simulink model "LMS_cs"  (R2023a)
settings: Solver=ode5  StartTime=0.0  StopTime=inf  FixedStep=1/200  RelTol=1e-3
PreLoadFcn:
  | mbxruntime.callbacks.PreLoadFcn(bdroot);
PostLoadFcn:
  | mbxruntime.callbacks.PostLoadFcn(bdroot);
InitFcn:
  | mbxruntime.callbacks.InitFcn(bdroot);
StartFcn:
  | mbxruntime.callbacks.StartFcn(bdroot);
StopFcn:
  | mbxruntime.callbacks.StopFcn(bdroot);
model workspace (MAT data in the model file):
  mbox_table : object (value not decoded)
  model_closed = 0
  sim_status = 0
undefined symbols (not defined in the file or in its folder): DiscIntNeverNeededParam, WheelL0, WheelL1, WheelR0, WheelR1
libraries: simulink x462, simulink_extras x117, PreScanSimulinkLibrary x33, PreScanUsefulBlocks x6, instrumentseriallib x5, simulink_need_slupdate x1
(part 6 of 68)

== system LMS_cs/WheelL0_BMW_X5_SUV_1 ==
  WheelL0_BMW_X5_SUV_1 : Inport  Tag=inport/JointActuator  OutDataTypeStr=Bus: PRESCAN_POSE_DATA  SampleTime=2/200  BusOutputAsStruct=on
  Actuator : Subsystem  Tag=VisuJoint  mask(PreScan Sink Block: VisuJoint){UniqueID=3662, Translate_ObjectID3D=BMW_X5_SUV_1.WheelL0, Rotate_ObjectID3D=BMW_X5_SUV_1.WheelL0, TimeStep=2/200, DisplayName=[]}
      mask prompts: UniqueID "Parent Unique ID"; Translate_ObjectID3D "Translate Object Name"; Rotate_ObjectID3D "Rotate Object Name"; TimeStep "Simulation Step"; DisplayName "Display Name"
      mask help:
      | The VisuJoint block provides a way to adapt the location and orientation of a part of an object.
      |
      | For more information, please click Help.
      settings: DeleteFcn=PreScanBlockDeleteFcn;
      mask Help: eval('openHelp(223)')
      mask Display: image(imread('Joint.png'))
  wires:
  WheelL0_BMW_X5_SUV_1/1 -> Actuator/1(Joint)

== system LMS_cs/WheelL0_BMW_X5_SUV_10 ==
  WheelL0_BMW_X5_SUV_10 : Inport  Tag=inport/JointActuator  OutDataTypeStr=Bus: PRESCAN_POSE_DATA  SampleTime=2/200  BusOutputAsStruct=on
  Actuator : Subsystem  Tag=VisuJoint  mask(PreScan Sink Block: VisuJoint){UniqueID=3671, Translate_ObjectID3D=BMW_X5_SUV_10.WheelL0, Rotate_ObjectID3D=BMW_X5_SUV_10.WheelL0, TimeStep=2/200, DisplayName=[]}
      mask prompts: UniqueID "Parent Unique ID"; Translate_ObjectID3D "Translate Object Name"; Rotate_ObjectID3D "Rotate Object Name"; TimeStep "Simulation Step"; DisplayName "Display Name"
      mask help:
      | The VisuJoint block provides a way to adapt the location and orientation of a part of an object.
      |
      | For more information, please click Help.
      settings: DeleteFcn=PreScanBlockDeleteFcn;
      mask Help: eval('openHelp(223)')
      mask Display: image(imread('Joint.png'))
  wires:
  WheelL0_BMW_X5_SUV_10/1 -> Actuator/1(Joint)

== system LMS_cs/WheelL0_BMW_X5_SUV_11 ==
  WheelL0_BMW_X5_SUV_11 : Inport  Tag=inport/JointActuator  OutDataTypeStr=Bus: PRESCAN_POSE_DATA  SampleTime=2/200  BusOutputAsStruct=on
  Actuator : Subsystem  Tag=VisuJoint  mask(PreScan Sink Block: VisuJoint){UniqueID=3672, Translate_ObjectID3D=BMW_X5_SUV_11.WheelL0, Rotate_ObjectID3D=BMW_X5_SUV_11.WheelL0, TimeStep=2/200, DisplayName=[]}
      mask prompts: UniqueID "Parent Unique ID"; Translate_ObjectID3D "Translate Object Name"; Rotate_ObjectID3D "Rotate Object Name"; TimeStep "Simulation Step"; DisplayName "Display Name"
      mask help:
      | The VisuJoint block provides a way to adapt the location and orientation of a part of an object.
      |
      | For more information, please click Help.
      settings: DeleteFcn=PreScanBlockDeleteFcn;
      mask Help: eval('openHelp(223)')
      mask Display: image(imread('Joint.png'))
  wires:
  WheelL0_BMW_X5_SUV_11/1 -> Actuator/1(Joint)

== system LMS_cs/WheelL0_BMW_X5_SUV_12 ==
  WheelL0_BMW_X5_SUV_12 : Inport  Tag=inport/JointActuator  OutDataTypeStr=Bus: PRESCAN_POSE_DATA  SampleTime=2/200  BusOutputAsStruct=on
  Actuator : Subsystem  Tag=VisuJoint  mask(PreScan Sink Block: VisuJoint){UniqueID=5321, Translate_ObjectID3D=BMW_X5_SUV_12.WheelL0, Rotate_ObjectID3D=BMW_X5_SUV_12.WheelL0, TimeStep=2/200, DisplayName=[]}
      mask prompts: UniqueID "Parent Unique ID"; Translate_ObjectID3D "Translate Object Name"; Rotate_ObjectID3D "Rotate Object Name"; TimeStep "Simulation Step"; DisplayName "Display Name"
      mask help:
      | The VisuJoint block provides a way to adapt the location and orientation of a part of an object.
      |
      | For more information, please click Help.
      settings: DeleteFcn=PreScanBlockDeleteFcn;
      mask Help: eval('openHelp(223)')
      mask Display: image(imread('Joint.png'))
  wires:
  WheelL0_BMW_X5_SUV_12/1 -> Actuator/1(Joint)

== system LMS_cs/WheelL0_BMW_X5_SUV_13 ==
  WheelL0_BMW_X5_SUV_13 : Inport  Tag=inport/JointActuator  OutDataTypeStr=Bus: PRESCAN_POSE_DATA  SampleTime=2/200  BusOutputAsStruct=on
  Actuator : Subsystem  Tag=VisuJoint  mask(PreScan Sink Block: VisuJoint){UniqueID=5322, Translate_ObjectID3D=BMW_X5_SUV_13.WheelL0, Rotate_ObjectID3D=BMW_X5_SUV_13.WheelL0, TimeStep=2/200, DisplayName=[]}
      mask prompts: UniqueID "Parent Unique ID"; Translate_ObjectID3D "Translate Object Name"; Rotate_ObjectID3D "Rotate Object Name"; TimeStep "Simulation Step"; DisplayName "Display Name"
      mask help:
      | The VisuJoint block provides a way to adapt the location and orientation of a part of an object.
      |
      | For more information, please click Help.
      settings: DeleteFcn=PreScanBlockDeleteFcn;
      mask Help: eval('openHelp(223)')
      mask Display: image(imread('Joint.png'))
  wires:
  WheelL0_BMW_X5_SUV_13/1 -> Actuator/1(Joint)

== system LMS_cs/WheelL0_BMW_X5_SUV_2 ==
  WheelL0_BMW_X5_SUV_2 : Inport  Tag=inport/JointActuator  OutDataTypeStr=Bus: PRESCAN_POSE_DATA  SampleTime=2/200  BusOutputAsStruct=on
  Actuator : Subsystem  Tag=VisuJoint  mask(PreScan Sink Block: VisuJoint){UniqueID=3663, Translate_ObjectID3D=BMW_X5_SUV_2.WheelL0, Rotate_ObjectID3D=BMW_X5_SUV_2.WheelL0, TimeStep=2/200, DisplayName=[]}
      mask prompts: UniqueID "Parent Unique ID"; Translate_ObjectID3D "Translate Object Name"; Rotate_ObjectID3D "Rotate Object Name"; TimeStep "Simulation Step"; DisplayName "Display Name"
      mask help:
      | The VisuJoint block provides a way to adapt the location and orientation of a part of an object.
      |
      | For more information, please click Help.
      settings: DeleteFcn=PreScanBlockDeleteFcn;
      mask Help: eval('openHelp(223)')
      mask Display: image(imread('Joint.png'))
  wires:
  WheelL0_BMW_X5_SUV_2/1 -> Actuator/1(Joint)

== system LMS_cs/WheelL0_BMW_X5_SUV_3 ==
  WheelL0_BMW_X5_SUV_3 : Inport  Tag=inport/JointActuator  OutDataTypeStr=Bus: PRESCAN_POSE_DATA  SampleTime=2/200  BusOutputAsStruct=on
  Actuator : Subsystem  Tag=VisuJoint  mask(PreScan Sink Block: VisuJoint){UniqueID=3664, Translate_ObjectID3D=BMW_X5_SUV_3.WheelL0, Rotate_ObjectID3D=BMW_X5_SUV_3.WheelL0, TimeStep=2/200, DisplayName=[]}
      mask prompts: UniqueID "Parent Unique ID"; Translate_ObjectID3D "Translate Object Name"; Rotate_ObjectID3D "Rotate Object Name"; TimeStep "Simulation Step"; DisplayName "Display Name"
      mask help:
      | The VisuJoint block provides a way to adapt the location and orientation of a part of an object.
      |
      | For more information, please click Help.
      settings: DeleteFcn=PreScanBlockDeleteFcn;
      mask Help: eval('openHelp(223)')
      mask Display: image(imread('Joint.png'))
  wires:
  WheelL0_BMW_X5_SUV_3/1 -> Actuator/1(Joint)

== system LMS_cs/WheelL0_BMW_X5_SUV_4 ==
  WheelL0_BMW_X5_SUV_4 : Inport  Tag=inport/JointActuator  OutDataTypeStr=Bus: PRESCAN_POSE_DATA  SampleTime=2/200  BusOutputAsStruct=on
  Actuator : Subsystem  Tag=VisuJoint  mask(PreScan Sink Block: VisuJoint){UniqueID=3665, Translate_ObjectID3D=BMW_X5_SUV_4.WheelL0, Rotate_ObjectID3D=BMW_X5_SUV_4.WheelL0, TimeStep=2/200, DisplayName=[]}
      mask prompts: UniqueID "Parent Unique ID"; Translate_ObjectID3D "Translate Object Name"; Rotate_ObjectID3D "Rotate Object Name"; TimeStep "Simulation Step"; DisplayName "Display Name"
      mask help:
      | The VisuJoint block provides a way to adapt the location and orientation of a part of an object.
      |
      | For more information, please click Help.
      settings: DeleteFcn=PreScanBlockDeleteFcn;
      mask Help: eval('openHelp(223)')
      mask Display: image(imread('Joint.png'))
  wires:
  WheelL0_BMW_X5_SUV_4/1 -> Actuator/1(Joint)

== system LMS_cs/WheelL0_BMW_X5_SUV_5 ==
  WheelL0_BMW_X5_SUV_5 : Inport  Tag=inport/JointActuator  OutDataTypeStr=Bus: PRESCAN_POSE_DATA  SampleTime=2/200  BusOutputAsStruct=on
  Actuator : Subsystem  Tag=VisuJoint  mask(PreScan Sink Block: VisuJoint){UniqueID=3666, Translate_ObjectID3D=BMW_X5_SUV_5.WheelL0, Rotate_ObjectID3D=BMW_X5_SUV_5.WheelL0, TimeStep=2/200, DisplayName=[]}
      mask prompts: UniqueID "Parent Unique ID"; Translate_ObjectID3D "Translate Object Name"; Rotate_ObjectID3D "Rotate Object Name"; TimeStep "Simulation Step"; DisplayName "Display Name"
      mask help:
      | The VisuJoint block provides a way to adapt the location and orientation of a part of an object.
      |
      | For more information, please click Help.
      settings: DeleteFcn=PreScanBlockDeleteFcn;
      mask Help: eval('openHelp(223)')
      mask Display: image(imread('Joint.png'))
  wires:
  WheelL0_BMW_X5_SUV_5/1 -> Actuator/1(Joint)

== system LMS_cs/WheelL0_BMW_X5_SUV_6 ==
  WheelL0_BMW_X5_SUV_6 : Inport  Tag=inport/JointActuator  OutDataTypeStr=Bus: PRESCAN_POSE_DATA  SampleTime=2/200  BusOutputAsStruct=on
  Actuator : Subsystem  Tag=VisuJoint  mask(PreScan Sink Block: VisuJoint){UniqueID=3667, Translate_ObjectID3D=BMW_X5_SUV_6.WheelL0, Rotate_ObjectID3D=BMW_X5_SUV_6.WheelL0, TimeStep=2/200, DisplayName=[]}
      mask prompts: UniqueID "Parent Unique ID"; Translate_ObjectID3D "Translate Object Name"; Rotate_ObjectID3D "Rotate Object Name"; TimeStep "Simulation Step"; DisplayName "Display Name"
      mask help:
      | The VisuJoint block provides a way to adapt the location and orientation of a part of an object.
      |
      | For more information, please click Help.
      settings: DeleteFcn=PreScanBlockDeleteFcn;
      mask Help: eval('openHelp(223)')
      mask Display: image(imread('Joint.png'))
  wires:
  WheelL0_BMW_X5_SUV_6/1 -> Actuator/1(Joint)

== system LMS_cs/WheelL0_BMW_X5_SUV_7 ==
  WheelL0_BMW_X5_SUV_7 : Inport  Tag=inport/JointActuator  OutDataTypeStr=Bus: PRESCAN_POSE_DATA  SampleTime=2/200  BusOutputAsStruct=on
  Actuator : Subsystem  Tag=VisuJoint  mask(PreScan Sink Block: VisuJoint){UniqueID=3668, Translate_ObjectID3D=BMW_X5_SUV_7.WheelL0, Rotate_ObjectID3D=BMW_X5_SUV_7.WheelL0, TimeStep=2/200, DisplayName=[]}
      mask prompts: UniqueID "Parent Unique ID"; Translate_ObjectID3D "Translate Object Name"; Rotate_ObjectID3D "Rotate Object Name"; TimeStep "Simulation Step"; DisplayName "Display Name"
      mask help:
      | The VisuJoint block provides a way to adapt the location and orientation of a part of an object.
      |
      | For more information, please click Help.
      settings: DeleteFcn=PreScanBlockDeleteFcn;
      mask Help: eval('openHelp(223)')
      mask Display: image(imread('Joint.png'))
  wires:
  WheelL0_BMW_X5_SUV_7/1 -> Actuator/1(Joint)

== system LMS_cs/WheelL0_BMW_X5_SUV_8 ==
  WheelL0_BMW_X5_SUV_8 : Inport  Tag=inport/JointActuator  OutDataTypeStr=Bus: PRESCAN_POSE_DATA  SampleTime=2/200  BusOutputAsStruct=on
  Actuator : Subsystem  Tag=VisuJoint  mask(PreScan Sink Block: VisuJoint){UniqueID=3669, Translate_ObjectID3D=BMW_X5_SUV_8.WheelL0, Rotate_ObjectID3D=BMW_X5_SUV_8.WheelL0, TimeStep=2/200, DisplayName=[]}
      mask prompts: UniqueID "Parent Unique ID"; Translate_ObjectID3D "Translate Object Name"; Rotate_ObjectID3D "Rotate Object Name"; TimeStep "Simulation Step"; DisplayName "Display Name"
      mask help:
      | The VisuJoint block provides a way to adapt the location and orientation of a part of an object.
      |
      | For more information, please click Help.
      settings: DeleteFcn=PreScanBlockDeleteFcn;
      mask Help: eval('openHelp(223)')
      mask Display: image(imread('Joint.png'))
  wires:
  WheelL0_BMW_X5_SUV_8/1 -> Actuator/1(Joint)

== system LMS_cs/WheelL0_BMW_X5_SUV_9 ==
  WheelL0_BMW_X5_SUV_9 : Inport  Tag=inport/JointActuator  OutDataTypeStr=Bus: PRESCAN_POSE_DATA  SampleTime=2/200  BusOutputAsStruct=on
  Actuator : Subsystem  Tag=VisuJoint  mask(PreScan Sink Block: VisuJoint){UniqueID=3670, Translate_ObjectID3D=BMW_X5_SUV_9.WheelL0, Rotate_ObjectID3D=BMW_X5_SUV_9.WheelL0, TimeStep=2/200, DisplayName=[]}
      mask prompts: UniqueID "Parent Unique ID"; Translate_ObjectID3D "Translate Object Name"; Rotate_ObjectID3D "Rotate Object Name"; TimeStep "Simulation Step"; DisplayName "Display Name"
      mask help:
      | The VisuJoint block provides a way to adapt the location and orientation of a part of an object.
      |
      | For more information, please click Help.
      settings: DeleteFcn=PreScanBlockDeleteFcn;
      mask Help: eval('openHelp(223)')
      mask Display: image(imread('Joint.png'))
  wires:
  WheelL0_BMW_X5_SUV_9/1 -> Actuator/1(Joint)

== system LMS_cs/WheelL1_Audi_A8_Sedan_1 ==
  WheelL1_Audi_A8_Sedan_1 : Inport  Tag=inport/JointActuator  OutDataTypeStr=Bus: PRESCAN_POSE_DATA  SampleTime=2/200  BusOutputAsStruct=on
  Actuator : Subsystem  Tag=VisuJoint  mask(PreScan Sink Block: VisuJoint){UniqueID=16, Translate_ObjectID3D=Audi_A8_Sedan_1.WheelL1, Rotate_ObjectID3D=Audi_A8_Sedan_1.WheelL1, TimeStep=2/200, DisplayName=[]}
      mask prompts: UniqueID "Parent Unique ID"; Translate_ObjectID3D "Translate Object Name"; Rotate_ObjectID3D "Rotate Object Name"; TimeStep "Simulation Step"; DisplayName "Display Name"
      mask help:
      | The VisuJoint block provides a way to adapt the location and orientation of a part of an object.
      |
      | For more information, please click Help.
      settings: DeleteFcn=PreScanBlockDeleteFcn;
      mask Help: eval('openHelp(223)')
      mask Display: image(imread('Joint.png'))
  wires:
  WheelL1_Audi_A8_Sedan_1/1 -> Actuator/1(Joint)

== system LMS_cs/WheelL1_BMW_X5_SUV_1 ==
  WheelL1_BMW_X5_SUV_1 : Inport  Tag=inport/JointActuator  OutDataTypeStr=Bus: PRESCAN_POSE_DATA  SampleTime=2/200  BusOutputAsStruct=on
  Actuator : Subsystem  Tag=VisuJoint  mask(PreScan Sink Block: VisuJoint){UniqueID=3662, Translate_ObjectID3D=BMW_X5_SUV_1.WheelL1, Rotate_ObjectID3D=BMW_X5_SUV_1.WheelL1, TimeStep=2/200, DisplayName=[]}
      mask prompts: UniqueID "Parent Unique ID"; Translate_ObjectID3D "Translate Object Name"; Rotate_ObjectID3D "Rotate Object Name"; TimeStep "Simulation Step"; DisplayName "Display Name"
      mask help:
      | The VisuJoint block provides a way to adapt the location and orientation of a part of an object.
      |
      | For more information, please click Help.
      settings: DeleteFcn=PreScanBlockDeleteFcn;
      mask Help: eval('openHelp(223)')
      mask Display: image(imread('Joint.png'))
  wires:
  WheelL1_BMW_X5_SUV_1/1 -> Actuator/1(Joint)

== system LMS_cs/WheelL1_BMW_X5_SUV_10 ==
  WheelL1_BMW_X5_SUV_10 : Inport  Tag=inport/JointActuator  OutDataTypeStr=Bus: PRESCAN_POSE_DATA  SampleTime=2/200  BusOutputAsStruct=on
  Actuator : Subsystem  Tag=VisuJoint  mask(PreScan Sink Block: VisuJoint){UniqueID=3671, Translate_ObjectID3D=BMW_X5_SUV_10.WheelL1, Rotate_ObjectID3D=BMW_X5_SUV_10.WheelL1, TimeStep=2/200, DisplayName=[]}
      mask prompts: UniqueID "Parent Unique ID"; Translate_ObjectID3D "Translate Object Name"; Rotate_ObjectID3D "Rotate Object Name"; TimeStep "Simulation Step"; DisplayName "Display Name"
      mask help:
      | The VisuJoint block provides a way to adapt the location and orientation of a part of an object.
      |
      | For more information, please click Help.
      settings: DeleteFcn=PreScanBlockDeleteFcn;
      mask Help: eval('openHelp(223)')
      mask Display: image(imread('Joint.png'))
  wires:
  WheelL1_BMW_X5_SUV_10/1 -> Actuator/1(Joint)

== system LMS_cs/WheelL1_BMW_X5_SUV_11 ==
  WheelL1_BMW_X5_SUV_11 : Inport  Tag=inport/JointActuator  OutDataTypeStr=Bus: PRESCAN_POSE_DATA  SampleTime=2/200  BusOutputAsStruct=on
  Actuator : Subsystem  Tag=VisuJoint  mask(PreScan Sink Block: VisuJoint){UniqueID=3672, Translate_ObjectID3D=BMW_X5_SUV_11.WheelL1, Rotate_ObjectID3D=BMW_X5_SUV_11.WheelL1, TimeStep=2/200, DisplayName=[]}
      mask prompts: UniqueID "Parent Unique ID"; Translate_ObjectID3D "Translate Object Name"; Rotate_ObjectID3D "Rotate Object Name"; TimeStep "Simulation Step"; DisplayName "Display Name"
      mask help:
      | The VisuJoint block provides a way to adapt the location and orientation of a part of an object.
      |
      | For more information, please click Help.
      settings: DeleteFcn=PreScanBlockDeleteFcn;
      mask Help: eval('openHelp(223)')
      mask Display: image(imread('Joint.png'))
  wires:
  WheelL1_BMW_X5_SUV_11/1 -> Actuator/1(Joint)

== system LMS_cs/WheelL1_BMW_X5_SUV_12 ==
  WheelL1_BMW_X5_SUV_12 : Inport  Tag=inport/JointActuator  OutDataTypeStr=Bus: PRESCAN_POSE_DATA  SampleTime=2/200  BusOutputAsStruct=on
  Actuator : Subsystem  Tag=VisuJoint  mask(PreScan Sink Block: VisuJoint){UniqueID=5321, Translate_ObjectID3D=BMW_X5_SUV_12.WheelL1, Rotate_ObjectID3D=BMW_X5_SUV_12.WheelL1, TimeStep=2/200, DisplayName=[]}
      mask prompts: UniqueID "Parent Unique ID"; Translate_ObjectID3D "Translate Object Name"; Rotate_ObjectID3D "Rotate Object Name"; TimeStep "Simulation Step"; DisplayName "Display Name"
      mask help:
      | The VisuJoint block provides a way to adapt the location and orientation of a part of an object.
      |
      | For more information, please click Help.
      settings: DeleteFcn=PreScanBlockDeleteFcn;
      mask Help: eval('openHelp(223)')
      mask Display: image(imread('Joint.png'))
  wires:
  WheelL1_BMW_X5_SUV_12/1 -> Actuator/1(Joint)

== system LMS_cs/WheelL1_BMW_X5_SUV_13 ==
  WheelL1_BMW_X5_SUV_13 : Inport  Tag=inport/JointActuator  OutDataTypeStr=Bus: PRESCAN_POSE_DATA  SampleTime=2/200  BusOutputAsStruct=on
  Actuator : Subsystem  Tag=VisuJoint  mask(PreScan Sink Block: VisuJoint){UniqueID=5322, Translate_ObjectID3D=BMW_X5_SUV_13.WheelL1, Rotate_ObjectID3D=BMW_X5_SUV_13.WheelL1, TimeStep=2/200, DisplayName=[]}
      mask prompts: UniqueID "Parent Unique ID"; Translate_ObjectID3D "Translate Object Name"; Rotate_ObjectID3D "Rotate Object Name"; TimeStep "Simulation Step"; DisplayName "Display Name"
      mask help:
      | The VisuJoint block provides a way to adapt the location and orientation of a part of an object.
      |
      | For more information, please click Help.
      settings: DeleteFcn=PreScanBlockDeleteFcn;
      mask Help: eval('openHelp(223)')
      mask Display: image(imread('Joint.png'))
  wires:
  WheelL1_BMW_X5_SUV_13/1 -> Actuator/1(Joint)

== system LMS_cs/WheelL1_BMW_X5_SUV_2 ==
  WheelL1_BMW_X5_SUV_2 : Inport  Tag=inport/JointActuator  OutDataTypeStr=Bus: PRESCAN_POSE_DATA  SampleTime=2/200  BusOutputAsStruct=on
  Actuator : Subsystem  Tag=VisuJoint  mask(PreScan Sink Block: VisuJoint){UniqueID=3663, Translate_ObjectID3D=BMW_X5_SUV_2.WheelL1, Rotate_ObjectID3D=BMW_X5_SUV_2.WheelL1, TimeStep=2/200, DisplayName=[]}
      mask prompts: UniqueID "Parent Unique ID"; Translate_ObjectID3D "Translate Object Name"; Rotate_ObjectID3D "Rotate Object Name"; TimeStep "Simulation Step"; DisplayName "Display Name"
      mask help:
      | The VisuJoint block provides a way to adapt the location and orientation of a part of an object.
      |
      | For more information, please click Help.
      settings: DeleteFcn=PreScanBlockDeleteFcn;
      mask Help: eval('openHelp(223)')
      mask Display: image(imread('Joint.png'))
  wires:
  WheelL1_BMW_X5_SUV_2/1 -> Actuator/1(Joint)

== system LMS_cs/WheelL1_BMW_X5_SUV_3 ==
  WheelL1_BMW_X5_SUV_3 : Inport  Tag=inport/JointActuator  OutDataTypeStr=Bus: PRESCAN_POSE_DATA  SampleTime=2/200  BusOutputAsStruct=on
  Actuator : Subsystem  Tag=VisuJoint  mask(PreScan Sink Block: VisuJoint){UniqueID=3664, Translate_ObjectID3D=BMW_X5_SUV_3.WheelL1, Rotate_ObjectID3D=BMW_X5_SUV_3.WheelL1, TimeStep=2/200, DisplayName=[]}
      mask prompts: UniqueID "Parent Unique ID"; Translate_ObjectID3D "Translate Object Name"; Rotate_ObjectID3D "Rotate Object Name"; TimeStep "Simulation Step"; DisplayName "Display Name"
      mask help:
      | The VisuJoint block provides a way to adapt the location and orientation of a part of an object.
      |
      | For more information, please click Help.
      settings: DeleteFcn=PreScanBlockDeleteFcn;
      mask Help: eval('openHelp(223)')
      mask Display: image(imread('Joint.png'))
  wires:
  WheelL1_BMW_X5_SUV_3/1 -> Actuator/1(Joint)

== system LMS_cs/WheelL1_BMW_X5_SUV_4 ==
  WheelL1_BMW_X5_SUV_4 : Inport  Tag=inport/JointActuator  OutDataTypeStr=Bus: PRESCAN_POSE_DATA  SampleTime=2/200  BusOutputAsStruct=on
  Actuator : Subsystem  Tag=VisuJoint  mask(PreScan Sink Block: VisuJoint){UniqueID=3665, Translate_ObjectID3D=BMW_X5_SUV_4.WheelL1, Rotate_ObjectID3D=BMW_X5_SUV_4.WheelL1, TimeStep=2/200, DisplayName=[]}
      mask prompts: UniqueID "Parent Unique ID"; Translate_ObjectID3D "Translate Object Name"; Rotate_ObjectID3D "Rotate Object Name"; TimeStep "Simulation Step"; DisplayName "Display Name"
      mask help:
      | The VisuJoint block provides a way to adapt the location and orientation of a part of an object.
      |
      | For more information, please click Help.
      settings: DeleteFcn=PreScanBlockDeleteFcn;
      mask Help: eval('openHelp(223)')
      mask Display: image(imread('Joint.png'))
  wires:
  WheelL1_BMW_X5_SUV_4/1 -> Actuator/1(Joint)

== system LMS_cs/WheelL1_BMW_X5_SUV_5 ==
  WheelL1_BMW_X5_SUV_5 : Inport  Tag=inport/JointActuator  OutDataTypeStr=Bus: PRESCAN_POSE_DATA  SampleTime=2/200  BusOutputAsStruct=on
  Actuator : Subsystem  Tag=VisuJoint  mask(PreScan Sink Block: VisuJoint){UniqueID=3666, Translate_ObjectID3D=BMW_X5_SUV_5.WheelL1, Rotate_ObjectID3D=BMW_X5_SUV_5.WheelL1, TimeStep=2/200, DisplayName=[]}
      mask prompts: UniqueID "Parent Unique ID"; Translate_ObjectID3D "Translate Object Name"; Rotate_ObjectID3D "Rotate Object Name"; TimeStep "Simulation Step"; DisplayName "Display Name"
      mask help:
      | The VisuJoint block provides a way to adapt the location and orientation of a part of an object.
      |
      | For more information, please click Help.
      settings: DeleteFcn=PreScanBlockDeleteFcn;
      mask Help: eval('openHelp(223)')
      mask Display: image(imread('Joint.png'))
  wires:
  WheelL1_BMW_X5_SUV_5/1 -> Actuator/1(Joint)

== system LMS_cs/WheelL1_BMW_X5_SUV_6 ==
  WheelL1_BMW_X5_SUV_6 : Inport  Tag=inport/JointActuator  OutDataTypeStr=Bus: PRESCAN_POSE_DATA  SampleTime=2/200  BusOutputAsStruct=on
  Actuator : Subsystem  Tag=VisuJoint  mask(PreScan Sink Block: VisuJoint){UniqueID=3667, Translate_ObjectID3D=BMW_X5_SUV_6.WheelL1, Rotate_ObjectID3D=BMW_X5_SUV_6.WheelL1, TimeStep=2/200, DisplayName=[]}
      mask prompts: UniqueID "Parent Unique ID"; Translate_ObjectID3D "Translate Object Name"; Rotate_ObjectID3D "Rotate Object Name"; TimeStep "Simulation Step"; DisplayName "Display Name"
      mask help:
      | The VisuJoint block provides a way to adapt the location and orientation of a part of an object.
      |
      | For more information, please click Help.
      settings: DeleteFcn=PreScanBlockDeleteFcn;
      mask Help: eval('openHelp(223)')
      mask Display: image(imread('Joint.png'))
  wires:
  WheelL1_BMW_X5_SUV_6/1 -> Actuator/1(Joint)

== system LMS_cs/WheelL1_BMW_X5_SUV_7 ==
  WheelL1_BMW_X5_SUV_7 : Inport  Tag=inport/JointActuator  OutDataTypeStr=Bus: PRESCAN_POSE_DATA  SampleTime=2/200  BusOutputAsStruct=on
  Actuator : Subsystem  Tag=VisuJoint  mask(PreScan Sink Block: VisuJoint){UniqueID=3668, Translate_ObjectID3D=BMW_X5_SUV_7.WheelL1, Rotate_ObjectID3D=BMW_X5_SUV_7.WheelL1, TimeStep=2/200, DisplayName=[]}
      mask prompts: UniqueID "Parent Unique ID"; Translate_ObjectID3D "Translate Object Name"; Rotate_ObjectID3D "Rotate Object Name"; TimeStep "Simulation Step"; DisplayName "Display Name"
      mask help:
      | The VisuJoint block provides a way to adapt the location and orientation of a part of an object.
      |
      | For more information, please click Help.
      settings: DeleteFcn=PreScanBlockDeleteFcn;
      mask Help: eval('openHelp(223)')
      mask Display: image(imread('Joint.png'))
  wires:
  WheelL1_BMW_X5_SUV_7/1 -> Actuator/1(Joint)

== system LMS_cs/WheelL1_BMW_X5_SUV_8 ==
  WheelL1_BMW_X5_SUV_8 : Inport  Tag=inport/JointActuator  OutDataTypeStr=Bus: PRESCAN_POSE_DATA  SampleTime=2/200  BusOutputAsStruct=on
  Actuator : Subsystem  Tag=VisuJoint  mask(PreScan Sink Block: VisuJoint){UniqueID=3669, Translate_ObjectID3D=BMW_X5_SUV_8.WheelL1, Rotate_ObjectID3D=BMW_X5_SUV_8.WheelL1, TimeStep=2/200, DisplayName=[]}
      mask prompts: UniqueID "Parent Unique ID"; Translate_ObjectID3D "Translate Object Name"; Rotate_ObjectID3D "Rotate Object Name"; TimeStep "Simulation Step"; DisplayName "Display Name"
      mask help:
      | The VisuJoint block provides a way to adapt the location and orientation of a part of an object.
      |
      | For more information, please click Help.
      settings: DeleteFcn=PreScanBlockDeleteFcn;
      mask Help: eval('openHelp(223)')
      mask Display: image(imread('Joint.png'))
  wires:
  WheelL1_BMW_X5_SUV_8/1 -> Actuator/1(Joint)

== system LMS_cs/WheelL1_BMW_X5_SUV_9 ==
  WheelL1_BMW_X5_SUV_9 : Inport  Tag=inport/JointActuator  OutDataTypeStr=Bus: PRESCAN_POSE_DATA  SampleTime=2/200  BusOutputAsStruct=on
  Actuator : Subsystem  Tag=VisuJoint  mask(PreScan Sink Block: VisuJoint){UniqueID=3670, Translate_ObjectID3D=BMW_X5_SUV_9.WheelL1, Rotate_ObjectID3D=BMW_X5_SUV_9.WheelL1, TimeStep=2/200, DisplayName=[]}
      mask prompts: UniqueID "Parent Unique ID"; Translate_ObjectID3D "Translate Object Name"; Rotate_ObjectID3D "Rotate Object Name"; TimeStep "Simulation Step"; DisplayName "Display Name"
      mask help:
      | The VisuJoint block provides a way to adapt the location and orientation of a part of an object.
      |
      | For more information, please click Help.
      settings: DeleteFcn=PreScanBlockDeleteFcn;
      mask Help: eval('openHelp(223)')
      mask Display: image(imread('Joint.png'))
  wires:
  WheelL1_BMW_X5_SUV_9/1 -> Actuator/1(Joint)

== system LMS_cs/WheelR0_Audi_A8_Sedan_1 ==
  WheelR0_Audi_A8_Sedan_1 : Inport  Tag=inport/JointActuator  OutDataTypeStr=Bus: PRESCAN_POSE_DATA  SampleTime=2/200  BusOutputAsStruct=on
  Actuator : Subsystem  Tag=VisuJoint  mask(PreScan Sink Block: VisuJoint){UniqueID=16, Translate_ObjectID3D=Audi_A8_Sedan_1.WheelR0, Rotate_ObjectID3D=Audi_A8_Sedan_1.WheelR0, TimeStep=2/200, DisplayName=[]}
      mask prompts: UniqueID "Parent Unique ID"; Translate_ObjectID3D "Translate Object Name"; Rotate_ObjectID3D "Rotate Object Name"; TimeStep "Simulation Step"; DisplayName "Display Name"
      mask help:
      | The VisuJoint block provides a way to adapt the location and orientation of a part of an object.
      |
      | For more information, please click Help.
      settings: DeleteFcn=PreScanBlockDeleteFcn;
      mask Help: eval('openHelp(223)')
      mask Display: image(imread('Joint.png'))
  wires:
  WheelR0_Audi_A8_Sedan_1/1 -> Actuator/1(Joint)

== system LMS_cs/WheelR0_BMW_X5_SUV_1 ==
  WheelR0_BMW_X5_SUV_1 : Inport  Tag=inport/JointActuator  OutDataTypeStr=Bus: PRESCAN_POSE_DATA  SampleTime=2/200  BusOutputAsStruct=on
  Actuator : Subsystem  Tag=VisuJoint  mask(PreScan Sink Block: VisuJoint){UniqueID=3662, Translate_ObjectID3D=BMW_X5_SUV_1.WheelR0, Rotate_ObjectID3D=BMW_X5_SUV_1.WheelR0, TimeStep=2/200, DisplayName=[]}
      mask prompts: UniqueID "Parent Unique ID"; Translate_ObjectID3D "Translate Object Name"; Rotate_ObjectID3D "Rotate Object Name"; TimeStep "Simulation Step"; DisplayName "Display Name"
      mask help:
      | The VisuJoint block provides a way to adapt the location and orientation of a part of an object.
      |
      | For more information, please click Help.
      settings: DeleteFcn=PreScanBlockDeleteFcn;
      mask Help: eval('openHelp(223)')
      mask Display: image(imread('Joint.png'))
  wires:
  WheelR0_BMW_X5_SUV_1/1 -> Actuator/1(Joint)

== system LMS_cs/WheelR0_BMW_X5_SUV_10 ==
  WheelR0_BMW_X5_SUV_10 : Inport  Tag=inport/JointActuator  OutDataTypeStr=Bus: PRESCAN_POSE_DATA  SampleTime=2/200  BusOutputAsStruct=on
  Actuator : Subsystem  Tag=VisuJoint  mask(PreScan Sink Block: VisuJoint){UniqueID=3671, Translate_ObjectID3D=BMW_X5_SUV_10.WheelR0, Rotate_ObjectID3D=BMW_X5_SUV_10.WheelR0, TimeStep=2/200, DisplayName=[]}
      mask prompts: UniqueID "Parent Unique ID"; Translate_ObjectID3D "Translate Object Name"; Rotate_ObjectID3D "Rotate Object Name"; TimeStep "Simulation Step"; DisplayName "Display Name"
      mask help:
      | The VisuJoint block provides a way to adapt the location and orientation of a part of an object.
      |
      | For more information, please click Help.
      settings: DeleteFcn=PreScanBlockDeleteFcn;
      mask Help: eval('openHelp(223)')
      mask Display: image(imread('Joint.png'))
  wires:
  WheelR0_BMW_X5_SUV_10/1 -> Actuator/1(Joint)

== system LMS_cs/WheelR0_BMW_X5_SUV_11 ==
  WheelR0_BMW_X5_SUV_11 : Inport  Tag=inport/JointActuator  OutDataTypeStr=Bus: PRESCAN_POSE_DATA  SampleTime=2/200  BusOutputAsStruct=on
  Actuator : Subsystem  Tag=VisuJoint  mask(PreScan Sink Block: VisuJoint){UniqueID=3672, Translate_ObjectID3D=BMW_X5_SUV_11.WheelR0, Rotate_ObjectID3D=BMW_X5_SUV_11.WheelR0, TimeStep=2/200, DisplayName=[]}
      mask prompts: UniqueID "Parent Unique ID"; Translate_ObjectID3D "Translate Object Name"; Rotate_ObjectID3D "Rotate Object Name"; TimeStep "Simulation Step"; DisplayName "Display Name"
      mask help:
      | The VisuJoint block provides a way to adapt the location and orientation of a part of an object.
      |
      | For more information, please click Help.
      settings: DeleteFcn=PreScanBlockDeleteFcn;
      mask Help: eval('openHelp(223)')
      mask Display: image(imread('Joint.png'))
  wires:
  WheelR0_BMW_X5_SUV_11/1 -> Actuator/1(Joint)

== system LMS_cs/WheelR0_BMW_X5_SUV_12 ==
  WheelR0_BMW_X5_SUV_12 : Inport  Tag=inport/JointActuator  OutDataTypeStr=Bus: PRESCAN_POSE_DATA  SampleTime=2/200  BusOutputAsStruct=on
  Actuator : Subsystem  Tag=VisuJoint  mask(PreScan Sink Block: VisuJoint){UniqueID=5321, Translate_ObjectID3D=BMW_X5_SUV_12.WheelR0, Rotate_ObjectID3D=BMW_X5_SUV_12.WheelR0, TimeStep=2/200, DisplayName=[]}
      mask prompts: UniqueID "Parent Unique ID"; Translate_ObjectID3D "Translate Object Name"; Rotate_ObjectID3D "Rotate Object Name"; TimeStep "Simulation Step"; DisplayName "Display Name"
      mask help:
      | The VisuJoint block provides a way to adapt the location and orientation of a part of an object.
      |
      | For more information, please click Help.
      settings: DeleteFcn=PreScanBlockDeleteFcn;
      mask Help: eval('openHelp(223)')
      mask Display: image(imread('Joint.png'))
  wires:
  WheelR0_BMW_X5_SUV_12/1 -> Actuator/1(Joint)

== system LMS_cs/WheelR0_BMW_X5_SUV_13 ==
  WheelR0_BMW_X5_SUV_13 : Inport  Tag=inport/JointActuator  OutDataTypeStr=Bus: PRESCAN_POSE_DATA  SampleTime=2/200  BusOutputAsStruct=on
  Actuator : Subsystem  Tag=VisuJoint  mask(PreScan Sink Block: VisuJoint){UniqueID=5322, Translate_ObjectID3D=BMW_X5_SUV_13.WheelR0, Rotate_ObjectID3D=BMW_X5_SUV_13.WheelR0, TimeStep=2/200, DisplayName=[]}
      mask prompts: UniqueID "Parent Unique ID"; Translate_ObjectID3D "Translate Object Name"; Rotate_ObjectID3D "Rotate Object Name"; TimeStep "Simulation Step"; DisplayName "Display Name"
      mask help:
      | The VisuJoint block provides a way to adapt the location and orientation of a part of an object.
      |
      | For more information, please click Help.
      settings: DeleteFcn=PreScanBlockDeleteFcn;
      mask Help: eval('openHelp(223)')
      mask Display: image(imread('Joint.png'))
  wires:
  WheelR0_BMW_X5_SUV_13/1 -> Actuator/1(Joint)

== system LMS_cs/WheelR0_BMW_X5_SUV_2 ==
  WheelR0_BMW_X5_SUV_2 : Inport  Tag=inport/JointActuator  OutDataTypeStr=Bus: PRESCAN_POSE_DATA  SampleTime=2/200  BusOutputAsStruct=on
  Actuator : Subsystem  Tag=VisuJoint  mask(PreScan Sink Block: VisuJoint){UniqueID=3663, Translate_ObjectID3D=BMW_X5_SUV_2.WheelR0, Rotate_ObjectID3D=BMW_X5_SUV_2.WheelR0, TimeStep=2/200, DisplayName=[]}
      mask prompts: UniqueID "Parent Unique ID"; Translate_ObjectID3D "Translate Object Name"; Rotate_ObjectID3D "Rotate Object Name"; TimeStep "Simulation Step"; DisplayName "Display Name"
      mask help:
      | The VisuJoint block provides a way to adapt the location and orientation of a part of an object.
      |
      | For more information, please click Help.
      settings: DeleteFcn=PreScanBlockDeleteFcn;
      mask Help: eval('openHelp(223)')
      mask Display: image(imread('Joint.png'))
  wires:
  WheelR0_BMW_X5_SUV_2/1 -> Actuator/1(Joint)

== system LMS_cs/WheelR0_BMW_X5_SUV_3 ==
  WheelR0_BMW_X5_SUV_3 : Inport  Tag=inport/JointActuator  OutDataTypeStr=Bus: PRESCAN_POSE_DATA  SampleTime=2/200  BusOutputAsStruct=on
  Actuator : Subsystem  Tag=VisuJoint  mask(PreScan Sink Block: VisuJoint){UniqueID=3664, Translate_ObjectID3D=BMW_X5_SUV_3.WheelR0, Rotate_ObjectID3D=BMW_X5_SUV_3.WheelR0, TimeStep=2/200, DisplayName=[]}
      mask prompts: UniqueID "Parent Unique ID"; Translate_ObjectID3D "Translate Object Name"; Rotate_ObjectID3D "Rotate Object Name"; TimeStep "Simulation Step"; DisplayName "Display Name"
      mask help:
      | The VisuJoint block provides a way to adapt the location and orientation of a part of an object.
      |
      | For more information, please click Help.
      settings: DeleteFcn=PreScanBlockDeleteFcn;
      mask Help: eval('openHelp(223)')
      mask Display: image(imread('Joint.png'))
  wires:
  WheelR0_BMW_X5_SUV_3/1 -> Actuator/1(Joint)

== system LMS_cs/WheelR0_BMW_X5_SUV_4 ==
  WheelR0_BMW_X5_SUV_4 : Inport  Tag=inport/JointActuator  OutDataTypeStr=Bus: PRESCAN_POSE_DATA  SampleTime=2/200  BusOutputAsStruct=on
  Actuator : Subsystem  Tag=VisuJoint  mask(PreScan Sink Block: VisuJoint){UniqueID=3665, Translate_ObjectID3D=BMW_X5_SUV_4.WheelR0, Rotate_ObjectID3D=BMW_X5_SUV_4.WheelR0, TimeStep=2/200, DisplayName=[]}
      mask prompts: UniqueID "Parent Unique ID"; Translate_ObjectID3D "Translate Object Name"; Rotate_ObjectID3D "Rotate Object Name"; TimeStep "Simulation Step"; DisplayName "Display Name"
      mask help:
      | The VisuJoint block provides a way to adapt the location and orientation of a part of an object.
      |
      | For more information, please click Help.
      settings: DeleteFcn=PreScanBlockDeleteFcn;
      mask Help: eval('openHelp(223)')
      mask Display: image(imread('Joint.png'))
  wires:
  WheelR0_BMW_X5_SUV_4/1 -> Actuator/1(Joint)

== system LMS_cs/WheelR0_BMW_X5_SUV_5 ==
  WheelR0_BMW_X5_SUV_5 : Inport  Tag=inport/JointActuator  OutDataTypeStr=Bus: PRESCAN_POSE_DATA  SampleTime=2/200  BusOutputAsStruct=on
  Actuator : Subsystem  Tag=VisuJoint  mask(PreScan Sink Block: VisuJoint){UniqueID=3666, Translate_ObjectID3D=BMW_X5_SUV_5.WheelR0, Rotate_ObjectID3D=BMW_X5_SUV_5.WheelR0, TimeStep=2/200, DisplayName=[]}
      mask prompts: UniqueID "Parent Unique ID"; Translate_ObjectID3D "Translate Object Name"; Rotate_ObjectID3D "Rotate Object Name"; TimeStep "Simulation Step"; DisplayName "Display Name"
      mask help:
      | The VisuJoint block provides a way to adapt the location and orientation of a part of an object.
      |
      | For more information, please click Help.
      settings: DeleteFcn=PreScanBlockDeleteFcn;
      mask Help: eval('openHelp(223)')
      mask Display: image(imread('Joint.png'))
  wires:
  WheelR0_BMW_X5_SUV_5/1 -> Actuator/1(Joint)

== system LMS_cs/WheelR0_BMW_X5_SUV_6 ==
  WheelR0_BMW_X5_SUV_6 : Inport  Tag=inport/JointActuator  OutDataTypeStr=Bus: PRESCAN_POSE_DATA  SampleTime=2/200  BusOutputAsStruct=on
  Actuator : Subsystem  Tag=VisuJoint  mask(PreScan Sink Block: VisuJoint){UniqueID=3667, Translate_ObjectID3D=BMW_X5_SUV_6.WheelR0, Rotate_ObjectID3D=BMW_X5_SUV_6.WheelR0, TimeStep=2/200, DisplayName=[]}
      mask prompts: UniqueID "Parent Unique ID"; Translate_ObjectID3D "Translate Object Name"; Rotate_ObjectID3D "Rotate Object Name"; TimeStep "Simulation Step"; DisplayName "Display Name"
      mask help:
      | The VisuJoint block provides a way to adapt the location and orientation of a part of an object.
      |
      | For more information, please click Help.
      settings: DeleteFcn=PreScanBlockDeleteFcn;
      mask Help: eval('openHelp(223)')
      mask Display: image(imread('Joint.png'))
  wires:
  WheelR0_BMW_X5_SUV_6/1 -> Actuator/1(Joint)

== system LMS_cs/WheelR0_BMW_X5_SUV_7 ==
  WheelR0_BMW_X5_SUV_7 : Inport  Tag=inport/JointActuator  OutDataTypeStr=Bus: PRESCAN_POSE_DATA  SampleTime=2/200  BusOutputAsStruct=on
  Actuator : Subsystem  Tag=VisuJoint  mask(PreScan Sink Block: VisuJoint){UniqueID=3668, Translate_ObjectID3D=BMW_X5_SUV_7.WheelR0, Rotate_ObjectID3D=BMW_X5_SUV_7.WheelR0, TimeStep=2/200, DisplayName=[]}
      mask prompts: UniqueID "Parent Unique ID"; Translate_ObjectID3D "Translate Object Name"; Rotate_ObjectID3D "Rotate Object Name"; TimeStep "Simulation Step"; DisplayName "Display Name"
      mask help:
      | The VisuJoint block provides a way to adapt the location and orientation of a part of an object.
      |
      | For more information, please click Help.
      settings: DeleteFcn=PreScanBlockDeleteFcn;
      mask Help: eval('openHelp(223)')
      mask Display: image(imread('Joint.png'))
  wires:
  WheelR0_BMW_X5_SUV_7/1 -> Actuator/1(Joint)

== system LMS_cs/WheelR0_BMW_X5_SUV_8 ==
  WheelR0_BMW_X5_SUV_8 : Inport  Tag=inport/JointActuator  OutDataTypeStr=Bus: PRESCAN_POSE_DATA  SampleTime=2/200  BusOutputAsStruct=on
  Actuator : Subsystem  Tag=VisuJoint  mask(PreScan Sink Block: VisuJoint){UniqueID=3669, Translate_ObjectID3D=BMW_X5_SUV_8.WheelR0, Rotate_ObjectID3D=BMW_X5_SUV_8.WheelR0, TimeStep=2/200, DisplayName=[]}
      mask prompts: UniqueID "Parent Unique ID"; Translate_ObjectID3D "Translate Object Name"; Rotate_ObjectID3D "Rotate Object Name"; TimeStep "Simulation Step"; DisplayName "Display Name"
      mask help:
      | The VisuJoint block provides a way to adapt the location and orientation of a part of an object.
      |
      | For more information, please click Help.
      settings: DeleteFcn=PreScanBlockDeleteFcn;
      mask Help: eval('openHelp(223)')
      mask Display: image(imread('Joint.png'))
  wires:
  WheelR0_BMW_X5_SUV_8/1 -> Actuator/1(Joint)

== system LMS_cs/WheelR0_BMW_X5_SUV_9 ==
  WheelR0_BMW_X5_SUV_9 : Inport  Tag=inport/JointActuator  OutDataTypeStr=Bus: PRESCAN_POSE_DATA  SampleTime=2/200  BusOutputAsStruct=on
  Actuator : Subsystem  Tag=VisuJoint  mask(PreScan Sink Block: VisuJoint){UniqueID=3670, Translate_ObjectID3D=BMW_X5_SUV_9.WheelR0, Rotate_ObjectID3D=BMW_X5_SUV_9.WheelR0, TimeStep=2/200, DisplayName=[]}
      mask prompts: UniqueID "Parent Unique ID"; Translate_ObjectID3D "Translate Object Name"; Rotate_ObjectID3D "Rotate Object Name"; TimeStep "Simulation Step"; DisplayName "Display Name"
      mask help:
      | The VisuJoint block provides a way to adapt the location and orientation of a part of an object.
      |
      | For more information, please click Help.
      settings: DeleteFcn=PreScanBlockDeleteFcn;
      mask Help: eval('openHelp(223)')
      mask Display: image(imread('Joint.png'))
  wires:
  WheelR0_BMW_X5_SUV_9/1 -> Actuator/1(Joint)

== system LMS_cs/WheelR1_Audi_A8_Sedan_1 ==
  WheelR1_Audi_A8_Sedan_1 : Inport  Tag=inport/JointActuator  OutDataTypeStr=Bus: PRESCAN_POSE_DATA  SampleTime=2/200  BusOutputAsStruct=on
  Actuator : Subsystem  Tag=VisuJoint  mask(PreScan Sink Block: VisuJoint){UniqueID=16, Translate_ObjectID3D=Audi_A8_Sedan_1.WheelR1, Rotate_ObjectID3D=Audi_A8_Sedan_1.WheelR1, TimeStep=2/200, DisplayName=[]}
      mask prompts: UniqueID "Parent Unique ID"; Translate_ObjectID3D "Translate Object Name"; Rotate_ObjectID3D "Rotate Object Name"; TimeStep "Simulation Step"; DisplayName "Display Name"
      mask help:
      | The VisuJoint block provides a way to adapt the location and orientation of a part of an object.
      |
      | For more information, please click Help.
      settings: DeleteFcn=PreScanBlockDeleteFcn;
      mask Help: eval('openHelp(223)')
      mask Display: image(imread('Joint.png'))
  wires:
  WheelR1_Audi_A8_Sedan_1/1 -> Actuator/1(Joint)

== system LMS_cs/WheelR1_BMW_X5_SUV_1 ==
  WheelR1_BMW_X5_SUV_1 : Inport  Tag=inport/JointActuator  OutDataTypeStr=Bus: PRESCAN_POSE_DATA  SampleTime=2/200  BusOutputAsStruct=on
  Actuator : Subsystem  Tag=VisuJoint  mask(PreScan Sink Block: VisuJoint){UniqueID=3662, Translate_ObjectID3D=BMW_X5_SUV_1.WheelR1, Rotate_ObjectID3D=BMW_X5_SUV_1.WheelR1, TimeStep=2/200, DisplayName=[]}
      mask prompts: UniqueID "Parent Unique ID"; Translate_ObjectID3D "Translate Object Name"; Rotate_ObjectID3D "Rotate Object Name"; TimeStep "Simulation Step"; DisplayName "Display Name"
      mask help:
      | The VisuJoint block provides a way to adapt the location and orientation of a part of an object.
      |
      | For more information, please click Help.
      settings: DeleteFcn=PreScanBlockDeleteFcn;
      mask Help: eval('openHelp(223)')
      mask Display: image(imread('Joint.png'))
  wires:
  WheelR1_BMW_X5_SUV_1/1 -> Actuator/1(Joint)

== system LMS_cs/WheelR1_BMW_X5_SUV_10 ==
  WheelR1_BMW_X5_SUV_10 : Inport  Tag=inport/JointActuator  OutDataTypeStr=Bus: PRESCAN_POSE_DATA  SampleTime=2/200  BusOutputAsStruct=on
  Actuator : Subsystem  Tag=VisuJoint  mask(PreScan Sink Block: VisuJoint){UniqueID=3671, Translate_ObjectID3D=BMW_X5_SUV_10.WheelR1, Rotate_ObjectID3D=BMW_X5_SUV_10.WheelR1, TimeStep=2/200, DisplayName=[]}
      mask prompts: UniqueID "Parent Unique ID"; Translate_ObjectID3D "Translate Object Name"; Rotate_ObjectID3D "Rotate Object Name"; TimeStep "Simulation Step"; DisplayName "Display Name"
      mask help:
      | The VisuJoint block provides a way to adapt the location and orientation of a part of an object.
      |
      | For more information, please click Help.
      settings: DeleteFcn=PreScanBlockDeleteFcn;
      mask Help: eval('openHelp(223)')
      mask Display: image(imread('Joint.png'))
  wires:
  WheelR1_BMW_X5_SUV_10/1 -> Actuator/1(Joint)

== system LMS_cs/WheelR1_BMW_X5_SUV_11 ==
  WheelR1_BMW_X5_SUV_11 : Inport  Tag=inport/JointActuator  OutDataTypeStr=Bus: PRESCAN_POSE_DATA  SampleTime=2/200  BusOutputAsStruct=on
  Actuator : Subsystem  Tag=VisuJoint  mask(PreScan Sink Block: VisuJoint){UniqueID=3672, Translate_ObjectID3D=BMW_X5_SUV_11.WheelR1, Rotate_ObjectID3D=BMW_X5_SUV_11.WheelR1, TimeStep=2/200, DisplayName=[]}
      mask prompts: UniqueID "Parent Unique ID"; Translate_ObjectID3D "Translate Object Name"; Rotate_ObjectID3D "Rotate Object Name"; TimeStep "Simulation Step"; DisplayName "Display Name"
      mask help:
      | The VisuJoint block provides a way to adapt the location and orientation of a part of an object.
      |
      | For more information, please click Help.
      settings: DeleteFcn=PreScanBlockDeleteFcn;
      mask Help: eval('openHelp(223)')
      mask Display: image(imread('Joint.png'))
  wires:
  WheelR1_BMW_X5_SUV_11/1 -> Actuator/1(Joint)

== system LMS_cs/WheelR1_BMW_X5_SUV_12 ==
  WheelR1_BMW_X5_SUV_12 : Inport  Tag=inport/JointActuator  OutDataTypeStr=Bus: PRESCAN_POSE_DATA  SampleTime=2/200  BusOutputAsStruct=on
  Actuator : Subsystem  Tag=VisuJoint  mask(PreScan Sink Block: VisuJoint){UniqueID=5321, Translate_ObjectID3D=BMW_X5_SUV_12.WheelR1, Rotate_ObjectID3D=BMW_X5_SUV_12.WheelR1, TimeStep=2/200, DisplayName=[]}
      mask prompts: UniqueID "Parent Unique ID"; Translate_ObjectID3D "Translate Object Name"; Rotate_ObjectID3D "Rotate Object Name"; TimeStep "Simulation Step"; DisplayName "Display Name"
      mask help:
      | The VisuJoint block provides a way to adapt the location and orientation of a part of an object.
      |
      | For more information, please click Help.
      settings: DeleteFcn=PreScanBlockDeleteFcn;
      mask Help: eval('openHelp(223)')
      mask Display: image(imread('Joint.png'))
  wires:
  WheelR1_BMW_X5_SUV_12/1 -> Actuator/1(Joint)

== system LMS_cs/WheelR1_BMW_X5_SUV_13 ==
  WheelR1_BMW_X5_SUV_13 : Inport  Tag=inport/JointActuator  OutDataTypeStr=Bus: PRESCAN_POSE_DATA  SampleTime=2/200  BusOutputAsStruct=on
  Actuator : Subsystem  Tag=VisuJoint  mask(PreScan Sink Block: VisuJoint){UniqueID=5322, Translate_ObjectID3D=BMW_X5_SUV_13.WheelR1, Rotate_ObjectID3D=BMW_X5_SUV_13.WheelR1, TimeStep=2/200, DisplayName=[]}
      mask prompts: UniqueID "Parent Unique ID"; Translate_ObjectID3D "Translate Object Name"; Rotate_ObjectID3D "Rotate Object Name"; TimeStep "Simulation Step"; DisplayName "Display Name"
      mask help:
      | The VisuJoint block provides a way to adapt the location and orientation of a part of an object.
      |
      | For more information, please click Help.
      settings: DeleteFcn=PreScanBlockDeleteFcn;
      mask Help: eval('openHelp(223)')
      mask Display: image(imread('Joint.png'))
  wires:
  WheelR1_BMW_X5_SUV_13/1 -> Actuator/1(Joint)

== system LMS_cs/WheelR1_BMW_X5_SUV_2 ==
  WheelR1_BMW_X5_SUV_2 : Inport  Tag=inport/JointActuator  OutDataTypeStr=Bus: PRESCAN_POSE_DATA  SampleTime=2/200  BusOutputAsStruct=on
  Actuator : Subsystem  Tag=VisuJoint  mask(PreScan Sink Block: VisuJoint){UniqueID=3663, Translate_ObjectID3D=BMW_X5_SUV_2.WheelR1, Rotate_ObjectID3D=BMW_X5_SUV_2.WheelR1, TimeStep=2/200, DisplayName=[]}
      mask prompts: UniqueID "Parent Unique ID"; Translate_ObjectID3D "Translate Object Name"; Rotate_ObjectID3D "Rotate Object Name"; TimeStep "Simulation Step"; DisplayName "Display Name"
      mask help:
      | The VisuJoint block provides a way to adapt the location and orientation of a part of an object.
      |
      | For more information, please click Help.
      settings: DeleteFcn=PreScanBlockDeleteFcn;
      mask Help: eval('openHelp(223)')
      mask Display: image(imread('Joint.png'))
  wires:
  WheelR1_BMW_X5_SUV_2/1 -> Actuator/1(Joint)

== system LMS_cs/WheelR1_BMW_X5_SUV_3 ==
  WheelR1_BMW_X5_SUV_3 : Inport  Tag=inport/JointActuator  OutDataTypeStr=Bus: PRESCAN_POSE_DATA  SampleTime=2/200  BusOutputAsStruct=on
  Actuator : Subsystem  Tag=VisuJoint  mask(PreScan Sink Block: VisuJoint){UniqueID=3664, Translate_ObjectID3D=BMW_X5_SUV_3.WheelR1, Rotate_ObjectID3D=BMW_X5_SUV_3.WheelR1, TimeStep=2/200, DisplayName=[]}
      mask prompts: UniqueID "Parent Unique ID"; Translate_ObjectID3D "Translate Object Name"; Rotate_ObjectID3D "Rotate Object Name"; TimeStep "Simulation Step"; DisplayName "Display Name"
      mask help:
      | The VisuJoint block provides a way to adapt the location and orientation of a part of an object.
      |
      | For more information, please click Help.
      settings: DeleteFcn=PreScanBlockDeleteFcn;
      mask Help: eval('openHelp(223)')
      mask Display: image(imread('Joint.png'))
  wires:
  WheelR1_BMW_X5_SUV_3/1 -> Actuator/1(Joint)

== system LMS_cs/WheelR1_BMW_X5_SUV_4 ==
  WheelR1_BMW_X5_SUV_4 : Inport  Tag=inport/JointActuator  OutDataTypeStr=Bus: PRESCAN_POSE_DATA  SampleTime=2/200  BusOutputAsStruct=on
  Actuator : Subsystem  Tag=VisuJoint  mask(PreScan Sink Block: VisuJoint){UniqueID=3665, Translate_ObjectID3D=BMW_X5_SUV_4.WheelR1, Rotate_ObjectID3D=BMW_X5_SUV_4.WheelR1, TimeStep=2/200, DisplayName=[]}
      mask prompts: UniqueID "Parent Unique ID"; Translate_ObjectID3D "Translate Object Name"; Rotate_ObjectID3D "Rotate Object Name"; TimeStep "Simulation Step"; DisplayName "Display Name"
      mask help:
      | The VisuJoint block provides a way to adapt the location and orientation of a part of an object.
      |
      | For more information, please click Help.
      settings: DeleteFcn=PreScanBlockDeleteFcn;
      mask Help: eval('openHelp(223)')
      mask Display: image(imread('Joint.png'))
  wires:
  WheelR1_BMW_X5_SUV_4/1 -> Actuator/1(Joint)

== system LMS_cs/WheelR1_BMW_X5_SUV_5 ==
  WheelR1_BMW_X5_SUV_5 : Inport  Tag=inport/JointActuator  OutDataTypeStr=Bus: PRESCAN_POSE_DATA  SampleTime=2/200  BusOutputAsStruct=on
  Actuator : Subsystem  Tag=VisuJoint  mask(PreScan Sink Block: VisuJoint){UniqueID=3666, Translate_ObjectID3D=BMW_X5_SUV_5.WheelR1, Rotate_ObjectID3D=BMW_X5_SUV_5.WheelR1, TimeStep=2/200, DisplayName=[]}
      mask prompts: UniqueID "Parent Unique ID"; Translate_ObjectID3D "Translate Object Name"; Rotate_ObjectID3D "Rotate Object Name"; TimeStep "Simulation Step"; DisplayName "Display Name"
      mask help:
      | The VisuJoint block provides a way to adapt the location and orientation of a part of an object.
      |
      | For more information, please click Help.
      settings: DeleteFcn=PreScanBlockDeleteFcn;
      mask Help: eval('openHelp(223)')
      mask Display: image(imread('Joint.png'))
  wires:
  WheelR1_BMW_X5_SUV_5/1 -> Actuator/1(Joint)

== system LMS_cs/WheelR1_BMW_X5_SUV_6 ==
  WheelR1_BMW_X5_SUV_6 : Inport  Tag=inport/JointActuator  OutDataTypeStr=Bus: PRESCAN_POSE_DATA  SampleTime=2/200  BusOutputAsStruct=on
  Actuator : Subsystem  Tag=VisuJoint  mask(PreScan Sink Block: VisuJoint){UniqueID=3667, Translate_ObjectID3D=BMW_X5_SUV_6.WheelR1, Rotate_ObjectID3D=BMW_X5_SUV_6.WheelR1, TimeStep=2/200, DisplayName=[]}
      mask prompts: UniqueID "Parent Unique ID"; Translate_ObjectID3D "Translate Object Name"; Rotate_ObjectID3D "Rotate Object Name"; TimeStep "Simulation Step"; DisplayName "Display Name"
      mask help:
      | The VisuJoint block provides a way to adapt the location and orientation of a part of an object.
      |
      | For more information, please click Help.
      settings: DeleteFcn=PreScanBlockDeleteFcn;
      mask Help: eval('openHelp(223)')
      mask Display: image(imread('Joint.png'))
  wires:
  WheelR1_BMW_X5_SUV_6/1 -> Actuator/1(Joint)

== system LMS_cs/WheelR1_BMW_X5_SUV_7 ==
  WheelR1_BMW_X5_SUV_7 : Inport  Tag=inport/JointActuator  OutDataTypeStr=Bus: PRESCAN_POSE_DATA  SampleTime=2/200  BusOutputAsStruct=on
  Actuator : Subsystem  Tag=VisuJoint  mask(PreScan Sink Block: VisuJoint){UniqueID=3668, Translate_ObjectID3D=BMW_X5_SUV_7.WheelR1, Rotate_ObjectID3D=BMW_X5_SUV_7.WheelR1, TimeStep=2/200, DisplayName=[]}
      mask prompts: UniqueID "Parent Unique ID"; Translate_ObjectID3D "Translate Object Name"; Rotate_ObjectID3D "Rotate Object Name"; TimeStep "Simulation Step"; DisplayName "Display Name"
      mask help:
      | The VisuJoint block provides a way to adapt the location and orientation of a part of an object.
      |
      | For more information, please click Help.
      settings: DeleteFcn=PreScanBlockDeleteFcn;
      mask Help: eval('openHelp(223)')
      mask Display: image(imread('Joint.png'))
  wires:
  WheelR1_BMW_X5_SUV_7/1 -> Actuator/1(Joint)

== system LMS_cs/WheelR1_BMW_X5_SUV_8 ==
  WheelR1_BMW_X5_SUV_8 : Inport  Tag=inport/JointActuator  OutDataTypeStr=Bus: PRESCAN_POSE_DATA  SampleTime=2/200  BusOutputAsStruct=on
  Actuator : Subsystem  Tag=VisuJoint  mask(PreScan Sink Block: VisuJoint){UniqueID=3669, Translate_ObjectID3D=BMW_X5_SUV_8.WheelR1, Rotate_ObjectID3D=BMW_X5_SUV_8.WheelR1, TimeStep=2/200, DisplayName=[]}
      mask prompts: UniqueID "Parent Unique ID"; Translate_ObjectID3D "Translate Object Name"; Rotate_ObjectID3D "Rotate Object Name"; TimeStep "Simulation Step"; DisplayName "Display Name"
      mask help:
      | The VisuJoint block provides a way to adapt the location and orientation of a part of an object.
      |
      | For more information, please click Help.
      settings: DeleteFcn=PreScanBlockDeleteFcn;
      mask Help: eval('openHelp(223)')
      mask Display: image(imread('Joint.png'))
  wires:
  WheelR1_BMW_X5_SUV_8/1 -> Actuator/1(Joint)
